simulink model "lab1_ex1"  (R2025b)
settings: Solver=VariableStepAuto  StartTime=0.0  StopTime=10.0  RelTol=1e-3

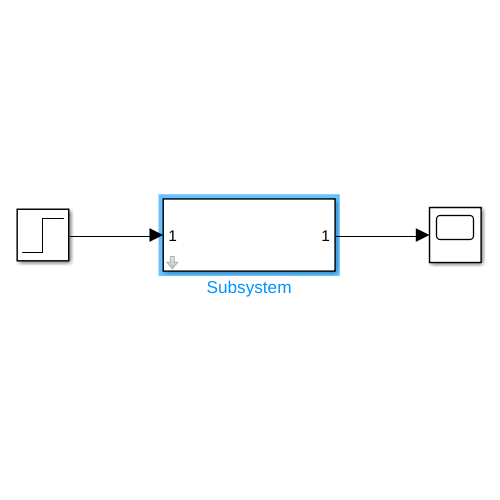
[thumbnail: Simulink's stored preview of the top-level diagram]
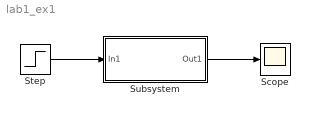
== system lab1_ex1 ==
  Scope : Scope
      settings: ActiveDisplayYMinimum=-0.12502155803746978  ActiveDisplayYMaximum=1.1251940223372283
  Step : Step  SampleTime=0
  Subsystem : Subsystem  mask{a=25}
      mask prompts: a "introdu a"
  wires:
  Step/1 -> Subsystem/1(In1)
  Subsystem/1(Out1) -> Scope/1

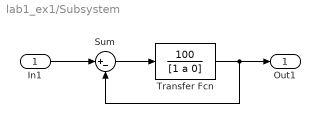
== system lab1_ex1/Subsystem ==
  In1 : Inport
  Sum : Sum  Inputs=|+-
  Transfer Fcn : TransferFcn  Numerator=[100]  Denominator=[1 a 0]
  Out1 : Outport
  wires:
  In1/1 -> Sum/1
  Transfer Fcn/1 -> Sum/2, Out1/1
  Sum/1 -> Transfer Fcn/1
